simulink model "control"  (R2024a)
settings: Solver=VariableStepAuto  StartTime=0.0  StopTime=10.0  RelTol=1e-3
settings Model: Creator=mustafaenesozdel  LastModifiedBy=mustafaenesozdel

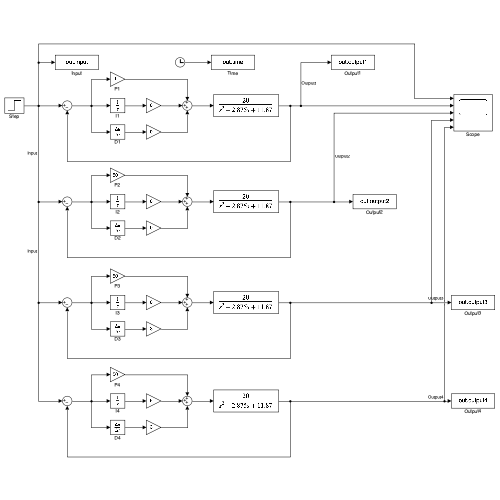
[thumbnail: Simulink's stored preview of the top-level diagram]
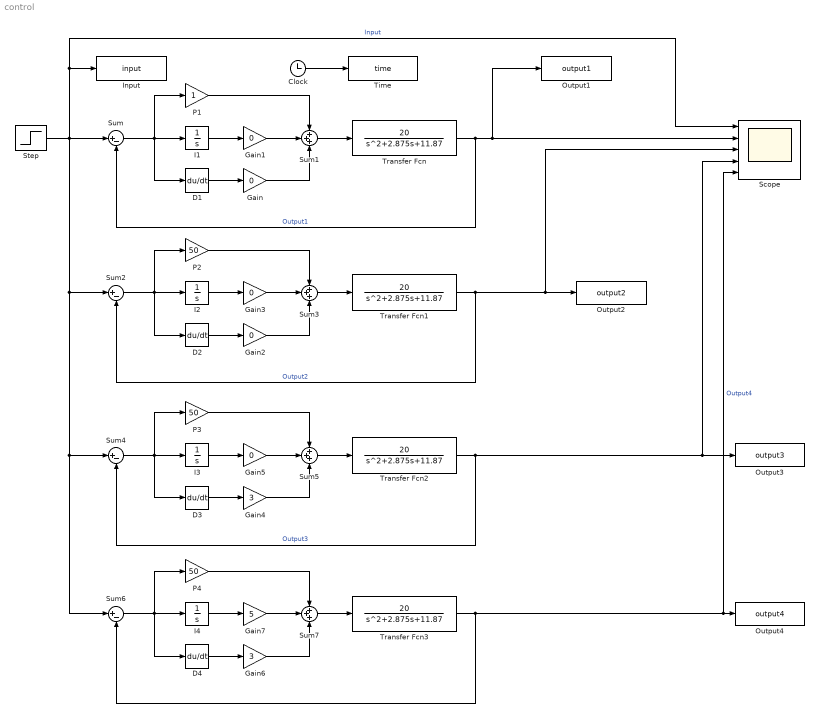
== system control ==
  Clock : Clock
  D{1..4} (4 alike) : Derivative
  Gain{,1..3,5} (5 alike) : Gain  Gain=0
  Gain4 : Gain  Gain=3
  Gain6 : Gain  Gain=3
  Gain7 : Gain  Gain=5
  I{1..4} (4 alike) : Integrator
  Input : ToWorkspace  VariableName=input  SaveFormat=Timeseries  SampleTime=-1
  Output1 : ToWorkspace  VariableName=output1  SaveFormat=Timeseries  SampleTime=-1
  Output2 : ToWorkspace  VariableName=output2  SaveFormat=Timeseries  SampleTime=-1
  Output3 : ToWorkspace  VariableName=output3  SaveFormat=Timeseries  SampleTime=-1
  Output4 : ToWorkspace  VariableName=output4  SaveFormat=Timeseries  SampleTime=-1
  P1 : Gain
  P2 : Gain  Gain=50
  P3 : Gain  Gain=50
  P4 : Gain  Gain=50
  Scope : Scope  NumInputPorts=5
  Step : Step  Time=0.0001  SampleTime=0
  Sum{,2,4,6} (4 alike) : Sum  Inputs=|+-
  Sum{1,3,5,7} (4 alike) : Sum  Inputs=+++
  Time : ToWorkspace  VariableName=time  SaveFormat=Timeseries  SampleTime=-1
  Transfer Fcn{,1..3} (4 alike) : TransferFcn  Numerator=[20]  Denominator=[1 2.875 11.87]
  wires:
  D1/1 -> Gain/1
  I1/1 -> Gain1/1
  Sum/1 -> I1/1, D1/1, P1/1
  P1/1 -> Sum1/1
  Gain/1 -> Sum1/3
  Gain1/1 -> Sum1/2
  Sum1/1 -> Transfer Fcn/1
  Transfer Fcn/1 -> Sum/2, Output1/1, Scope/2  "Output1"
  Sum3/1 -> Transfer Fcn1/1
  Gain3/1 -> Sum3/2
  D2/1 -> Gain2/1
  Transfer Fcn1/1 -> Scope/3, Output2/1, Sum2/2  "Output2"
  I2/1 -> Gain3/1
  Gain2/1 -> Sum3/3
  Sum2/1 -> I2/1, D2/1, P2/1
  P2/1 -> Sum3/1
  Clock/1 -> Time/1
  Sum5/1 -> Transfer Fcn2/1
  Gain5/1 -> Sum5/2
  Step/1 -> Scope/1, Input/1, Sum6/1, Sum4/1, Sum2/1, Sum/1  "Input"
  I3/1 -> Gain5/1
  P3/1 -> Sum5/1
  D3/1 -> Gain4/1
  Transfer Fcn2/1 -> Scope/4, Output3/1, Sum4/2  "Output3"
  Gain4/1 -> Sum5/3
  Sum4/1 -> I3/1, D3/1, P3/1
  Transfer Fcn3/1 -> Scope/5, Output4/1, Sum6/2  "Output4"
  Gain7/1 -> Sum7/2
  Gain6/1 -> Sum7/3
  P4/1 -> Sum7/1
  Sum6/1 -> I4/1, D4/1, P4/1
  Sum7/1 -> Transfer Fcn3/1
  I4/1 -> Gain7/1
  D4/1 -> Gain6/1
